simulink model "Astrobee_Sim"  (R2019b)
settings: Solver=VariableStepAuto  StartTime=0.0  StopTime=10.0  RelTol=1e-3
libraries: cstblocks x18
settings Model: Creator=abhi  LastModifiedBy=abhi

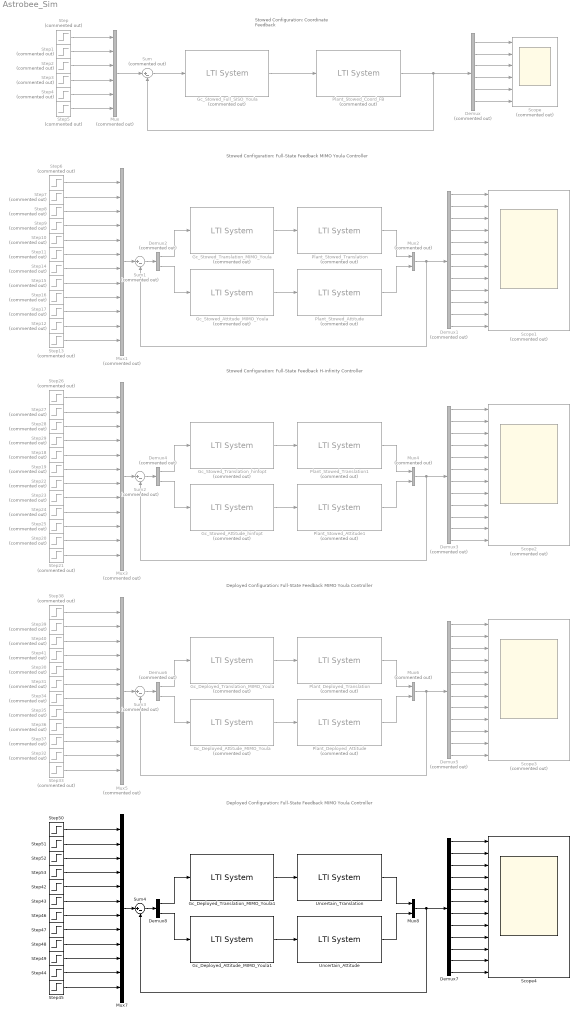
== system Astrobee_Sim ==
  note: Stowed Configuration:
      | Coordinate Feedback
  note: Stowed Configuration:
      | Full-State Feedback
      |
      | MIMO Youla Controller
  note: Stowed Configuration:
      | Full-State Feedback
      |
      | H-infinity Controller
  note: Deployed Configuration:
      | Full-State Feedback
      |
      | MIMO Youla Controller
  note: Deployed Configuration:
      | Full-State Feedback
      |
      | MIMO Youla Controller
  Demux : Demux  Commented=on  Outputs=6
  Demux1 : Demux  Commented=on  Outputs=12
  Demux2 : Demux  Commented=on  Outputs=2
  Demux3 : Demux  Commented=on  Outputs=12
  Demux4 : Demux  Commented=on  Outputs=2
  Demux5 : Demux  Commented=on  Outputs=12
  Demux6 : Demux  Commented=on  Outputs=2
  Demux7 : Demux  Outputs=12
  Demux8 : Demux  Outputs=2
  Gc_Deployed_Attitude_MIMO_Youla : cstblocks/LTI System  Commented=on  sys=Gc_Deployed_Attitude_MIMO_Youla  IC=[]
  Gc_Deployed_Attitude_MIMO_Youla1 : cstblocks/LTI System  sys=Gc_Deployed_Attitude_MIMO_Youla  IC=[]
  Gc_Deployed_Translation_MIMO_Youla : cstblocks/LTI System  Commented=on  sys=Gc_Deployed_Translation_MIMO_Youla  IC=[]
  Gc_Deployed_Translation_MIMO_Youla1 : cstblocks/LTI System  sys=Gc_Deployed_Translation_MIMO_Youla  IC=[]
  Gc_Stowed_Attitude_MIMO_Youla : cstblocks/LTI System  Commented=on  sys=Gc_Stowed_Attitude_MIMO_Youla  IC=[]
  Gc_Stowed_Attitude_hinfopt : cstblocks/LTI System  Commented=on  sys=Gc_Stowed_Attitude_hinfopt  IC=[]
  Gc_Stowed_Full_SISO_Youla : cstblocks/LTI System  Commented=on  sys=Gc_Stowed_Full_SISO_Youla  IC=[]
  Gc_Stowed_Translation_MIMO_Youla : cstblocks/LTI System  Commented=on  sys=Gc_Stowed_Translation_MIMO_Youla  IC=[]
  Gc_Stowed_Translation_hinfopt : cstblocks/LTI System  Commented=on  sys=Gc_Stowed_Translation_hinfopt  IC=[]
  Mux : Mux  Commented=on  Inputs=6
  Mux1 : Mux  Commented=on  Inputs=12
  Mux2 : Mux  Commented=on  Inputs=2
  Mux3 : Mux  Commented=on  Inputs=12
  Mux4 : Mux  Commented=on  Inputs=2
  Mux5 : Mux  Commented=on  Inputs=12
  Mux6 : Mux  Commented=on  Inputs=2
  Mux7 : Mux  Inputs=12
  Mux8 : Mux  Inputs=2
  Plant_Deployed_Attitude : cstblocks/LTI System  Commented=on  sys=Plant_Deployed_Attitude  IC=[]
  Plant_Deployed_Translation : cstblocks/LTI System  Commented=on  sys=Plant_Deployed_Translation  IC=[]
  Plant_Stowed_Attitude : cstblocks/LTI System  Commented=on  sys=Plant_Stowed_Attitude  IC=[]
  Plant_Stowed_Attitude1 : cstblocks/LTI System  Commented=on  sys=Plant_Stowed_Attitude  IC=[]
  Plant_Stowed_Coord_FB : cstblocks/LTI System  Commented=on  sys=Plant_Stowed_Coord_FB  IC=[]
  Plant_Stowed_Translation : cstblocks/LTI System  Commented=on  sys=Plant_Stowed_Translation  IC=[]
  Plant_Stowed_Translation1 : cstblocks/LTI System  Commented=on  sys=Plant_Stowed_Translation  IC=[]
  Scope : Scope  Commented=on  NumInputPorts=6
  Scope1 : Scope  Commented=on  NumInputPorts=12
  Scope2 : Scope  Commented=on  NumInputPorts=12
  Scope3 : Scope  Commented=on  NumInputPorts=12
  Scope4 : Scope  NumInputPorts=12
  Step{,1..41} (42 alike) : Step  Commented=on  SampleTime=0
  Step{42..53} (12 alike) : Step  SampleTime=0
  Sum{,1..3} (4 alike) : Sum  Commented=on  Inputs=|+-
  Sum4 : Sum  Inputs=|+-
  Uncertain_Attitude : cstblocks/LTI System  sys=Uncertain_Attitude  IC=[]
  Uncertain_Translation : cstblocks/LTI System  sys=Uncertain_Translation  IC=[]
  wires:
  Gc_Stowed_Full_SISO_Youla/1 -> Plant_Stowed_Coord_FB/1
  Plant_Stowed_Coord_FB/1 -> Sum/2, Demux/1
  Sum/1 -> Gc_Stowed_Full_SISO_Youla/1
  Mux/1 -> Sum/1
  Step/1 -> Mux/1
  Step1/1 -> Mux/2
  Step4/1 -> Mux/5
  Step5/1 -> Mux/6
  Step3/1 -> Mux/4
  Step2/1 -> Mux/3
  Demux/1 -> Scope/1
  Demux/2 -> Scope/2
  Demux/3 -> Scope/3
  Demux/4 -> Scope/4
  Demux/5 -> Scope/5
  Demux/6 -> Scope/6
  Demux1/3 -> Scope1/3
  Step6/1 -> Mux1/1
  Step10/1 -> Mux1/5
  Mux2/1 -> Demux1/1, Sum1/2
  Step11/1 -> Mux1/6
  Step8/1 -> Mux1/3
  Step9/1 -> Mux1/4
  Step7/1 -> Mux1/2
  Demux1/5 -> Scope1/5
  Demux1/2 -> Scope1/2
  Demux1/4 -> Scope1/4
  Demux1/6 -> Scope1/6
  Demux1/1 -> Scope1/1
  Demux2/1 -> Gc_Stowed_Translation_MIMO_Youla/1
  Demux2/2 -> Gc_Stowed_Attitude_MIMO_Youla/1
  Sum1/1 -> Demux2/1
  Step14/1 -> Mux1/7
  Step12/1 -> Mux1/11
  Step13/1 -> Mux1/12
  Step16/1 -> Mux1/9
  Step17/1 -> Mux1/10
  Demux1/7 -> Scope1/7
  Demux1/8 -> Scope1/8
  Demux1/9 -> Scope1/9
  Demux1/10 -> Scope1/10
  Demux1/11 -> Scope1/11
  Demux1/12 -> Scope1/12
  Mux1/1 -> Sum1/1
  Step15/1 -> Mux1/8
  Gc_Stowed_Translation_MIMO_Youla/1 -> Plant_Stowed_Translation/1
  Gc_Stowed_Attitude_MIMO_Youla/1 -> Plant_Stowed_Attitude/1
  Plant_Stowed_Translation/1 -> Mux2/1
  Plant_Stowed_Attitude/1 -> Mux2/2
  Step22/1 -> Mux3/7
  Demux3/9 -> Scope2/9
  Demux3/10 -> Scope2/10
  Step25/1 -> Mux3/10
  Step26/1 -> Mux3/1
  Mux4/1 -> Demux3/1, Sum2/2
  Demux4/2 -> Gc_Stowed_Attitude_hinfopt/1
  Demux3/4 -> Scope2/4
  Plant_Stowed_Attitude1/1 -> Mux4/2
  Demux3/1 -> Scope2/1
  Step18/1 -> Mux3/5
  Demux3/11 -> Scope2/11
  Step28/1 -> Mux3/3
  Demux3/5 -> Scope2/5
  Demux3/3 -> Scope2/3
  Demux3/8 -> Scope2/8
  Step21/1 -> Mux3/12
  Step24/1 -> Mux3/9
  Step29/1 -> Mux3/4
  Demux3/7 -> Scope2/7
  Step20/1 -> Mux3/11
  Demux3/2 -> Scope2/2
  Plant_Stowed_Translation1/1 -> Mux4/1
  Demux3/6 -> Scope2/6
  Step19/1 -> Mux3/6
  Demux3/12 -> Scope2/12
  Gc_Stowed_Translation_hinfopt/1 -> Plant_Stowed_Translation1/1
  Gc_Stowed_Attitude_hinfopt/1 -> Plant_Stowed_Attitude1/1
  Step23/1 -> Mux3/8
  Step27/1 -> Mux3/2
  Sum2/1 -> Demux4/1
  Demux4/1 -> Gc_Stowed_Translation_hinfopt/1
  Mux3/1 -> Sum2/1
  Sum3/1 -> Demux6/1
  Plant_Deployed_Attitude/1 -> Mux6/2
  Gc_Deployed_Attitude_MIMO_Youla/1 -> Plant_Deployed_Attitude/1
  Demux5/8 -> Scope3/8
  Step30/1 -> Mux5/5
  Demux6/1 -> Gc_Deployed_Translation_MIMO_Youla/1
  Demux6/2 -> Gc_Deployed_Attitude_MIMO_Youla/1
  Demux5/11 -> Scope3/11
  Demux5/10 -> Scope3/10
  Step36/1 -> Mux5/9
  Step41/1 -> Mux5/4
  Mux5/1 -> Sum3/1
  Demux5/2 -> Scope3/2
  Step37/1 -> Mux5/10
  Mux6/1 -> Demux5/1, Sum3/2
  Demux5/12 -> Scope3/12
  Plant_Deployed_Translation/1 -> Mux6/1
  Step34/1 -> Mux5/7
  Step39/1 -> Mux5/2
  Step40/1 -> Mux5/3
  Demux5/1 -> Scope3/1
  Step33/1 -> Mux5/12
  Demux5/7 -> Scope3/7
  Demux5/5 -> Scope3/5
  Gc_Deployed_Translation_MIMO_Youla/1 -> Plant_Deployed_Translation/1
  Demux5/9 -> Scope3/9
  Demux5/6 -> Scope3/6
  Step31/1 -> Mux5/6
  Step38/1 -> Mux5/1
  Step35/1 -> Mux5/8
  Demux5/4 -> Scope3/4
  Demux5/3 -> Scope3/3
  Step32/1 -> Mux5/11
  Demux7/11 -> Scope4/11
  Demux7/3 -> Scope4/3
  Step44/1 -> Mux7/11
  Step43/1 -> Mux7/6
  Step47/1 -> Mux7/8
  Demux7/12 -> Scope4/12
  Demux7/4 -> Scope4/4
  Demux7/9 -> Scope4/9
  Gc_Deployed_Attitude_MIMO_Youla1/1 -> Uncertain_Attitude/1
  Sum4/1 -> Demux8/1
  Demux8/2 -> Gc_Deployed_Attitude_MIMO_Youla1/1
  Step49/1 -> Mux7/10
  Step42/1 -> Mux7/5
  Demux7/7 -> Scope4/7
  Demux8/1 -> Gc_Deployed_Translation_MIMO_Youla1/1
  Step50/1 -> Mux7/1
  Step48/1 -> Mux7/9
  Step53/1 -> Mux7/4
  Mux7/1 -> Sum4/1
  Demux7/8 -> Scope4/8
  Uncertain_Attitude/1 -> Mux8/2
  Demux7/2 -> Scope4/2
  Gc_Deployed_Translation_MIMO_Youla1/1 -> Uncertain_Translation/1
  Mux8/1 -> Demux7/1, Sum4/2
  Demux7/10 -> Scope4/10
  Uncertain_Translation/1 -> Mux8/1
  Step46/1 -> Mux7/7
  Step51/1 -> Mux7/2
  Step52/1 -> Mux7/3
  Demux7/1 -> Scope4/1
  Step45/1 -> Mux7/12
  Demux7/5 -> Scope4/5
  Demux7/6 -> Scope4/6
